simulink library "lib_controller"  (R2015a)
settings: Solver=ode45  StartTime=0.0  StopTime=10.0  RelTol=1e-3
values from neighbouring files (symbols this model uses):
  CG_0 = [0,0,0.02]'    [SetupComplete.m]
  g = 9.81    [SetupComplete.m]
  h_M = 0.064    [SetupComplete.m]
  I_BAC_0 = [ Ix,0,Ixz;0,Iy,0;Ixz,0,Iz]    [SetupComplete.m]
  l = 0.3450    (= 0.345)    [NDI_components.m]    (also in SetupComplete.m; robust_controller.m)
  m = 3.51    [SetupComplete.m]
  m_0 = 2.61    [SetupComplete.m]
  m_M = 0.300    (= 0.3)    [SetupComplete.m]
  T_sim = 0.01    [Run3Copter.m]
undefined symbols (not defined in the file or in its folder): Theta_1_roll_last, Theta_2_roll_last, Theta_3_roll_last, V_long_lastA_w_z, V_long_lastAoA, V_roll_last, V_yaw_last, W_long_lastA_w_z, W_long_lastAoA, W_roll_last, W_yaw_last
libraries: simulink x65, Adaptive_FaultTolerantControl x8, lib_controller x5, qcatlib x4, dspinverses x4, aerolibtransform2 x3, aerolib6dofsys x1
(part 10 of 10)

== matlab function lib_controller/Controller/NDI+CA Controller/9DOF ANN+NDI+CA Controller - No massic update/F(X) 9DOF_UVWPQR ==
  data: fx output size=[6,1]; prev_input input size=[9,1]; gforce_body input size=[3,1]; omega_body input size=[3,1]; v_body input size=[3,1]
function fx = fx(prev_input, gforce_body, omega_body, v_body)
    % Calculates f_hat(x). The expression is calculated in NDI_components
    % x_dot = f(x) + g(x,u)
    %   g(x,u) ~= g(x,u0) + jac(g(x,u), u)(u0) * (u - u0)
    %   g(x,u) ~= h(x,u0) + jac(g(x,u), u)(u0) * u
    % x_dot = f_hat(x) + jac(g(x,u), u) * u
    %   f_hat(x) = f(x) + g(x,u0) - jac(g(x,u), u)(u0) *  u0
    %   g_hat(x) = jac(g(x,u), u)(u0)
    % x_dot = f_hat(x) + g_hat(x) * u
    tau1_0 = prev_input(1);
    eta1_0 = prev_input(2);
    gamma1_0 = prev_input(3);
    tau2_0 = prev_input(4);
    eta2_0 = prev_input(5);
    gamma2_0 = prev_input(6);
    tau3_0 = prev_input(7);
    eta3_0 = prev_input(8);
    gamma3_0 = prev_input(9);
    Gx =  gforce_body(1);
    Gy =  gforce_body(2);
    Gz =  gforce_body(3);
    U = v_body(1);
    V = v_body(2);
    W = v_body(3);
    P = omega_body(1);
    Q = omega_body(2);
    R = omega_body(3);

    % This matrix was precomputed in NDI_components.m
    % TODO Precompute sines and cosines to improve performance. Some
    % repeated terms can also be precomputed
    
 fx = [...
 5.88e-5*P^2 + 0.00285*P*R - 5.88e-5*R^2 + 1.0*V*R + 0.285*Gx - 1.0*Q*W + 4.27*gamma1_0*tau1_0*cos(gamma1_0) + 5.14e-4*gamma2_0*tau2_0*cos(gamma2_0) + 5.14e-4*gamma3_0*tau3_0*cos(gamma3_0) - 5.14e-4*eta1_0*tau1_0*cos(eta1_0)*cos(gamma1_0) + 4.27*eta2_0*tau2_0*cos(eta2_0)*cos(gamma2_0) + 4.27*eta3_0*tau3_0*cos(eta3_0)*cos(gamma3_0) + 0.038*eta1_0*tau1_0*cos(gamma1_0)*sin(eta1_0) - 0.019*eta2_0*tau2_0*cos(gamma2_0)*sin(eta2_0) - 0.019*eta3_0*tau3_0*cos(gamma3_0)*sin(eta3_0) + 0.038*gamma1_0*tau1_0*cos(eta1_0)*sin(gamma1_0) - 0.019*gamma2_0*tau2_0*cos(eta2_0)*sin(gamma2_0) - 0.019*gamma3_0*tau3_0*cos(eta3_0)*sin(gamma3_0) + 5.14e-4*gamma1_0*tau1_0*sin(eta1_0)*sin(gamma1_0) - 4.27*gamma2_0*tau2_0*sin(eta2_0)*sin(gamma2_0) - 4.27*gamma3_0*tau3_0*sin(eta3_0)*sin(gamma3_0);
        0.285*Gy + 6.54e-5*P*Q + 0.00281*Q*R + 1.0*P*W - 1.0*R*U - 6.56e-4*gamma1_0*tau1_0*cos(gamma1_0) - 4.27*gamma2_0*tau2_0*cos(gamma2_0) - 4.27*gamma3_0*tau3_0*cos(gamma3_0) - 4.27*eta1_0*tau1_0*cos(eta1_0)*cos(gamma1_0) - 3.21e-4*eta2_0*tau2_0*cos(eta2_0)*cos(gamma2_0) + 0.00163*eta3_0*tau3_0*cos(eta3_0)*cos(gamma3_0) - 1.53e-5*eta1_0*tau1_0*cos(gamma1_0)*sin(eta1_0) + 0.042*eta2_0*tau2_0*cos(gamma2_0)*sin(eta2_0) - 0.042*eta3_0*tau3_0*cos(gamma3_0)*sin(eta3_0) - 1.53e-5*gamma1_0*tau1_0*cos(eta1_0)*sin(gamma1_0) + 0.042*gamma2_0*tau2_0*cos(eta2_0)*sin(gamma2_0) - 0.042*gamma3_0*tau3_0*cos(eta3_0)*sin(gamma3_0) + 4.27*gamma1_0*tau1_0*sin(eta1_0)*sin(gamma1_0) + 3.21e-4*gamma2_0*tau2_0*sin(eta2_0)*sin(gamma2_0) - 0.00163*gamma3_0*tau3_0*sin(eta3_0)*sin(gamma3_0);
                                                                                                                                                                                                                                                                                                                                                                                                                                                - 0.0015*P^2 - 1.0*V*P - 0.0015*Q^2 + 1.0*U*Q + 0.285*Gz - 4.27*eta1_0*tau1_0*cos(gamma1_0)*sin(eta1_0) - 4.27*eta2_0*tau2_0*cos(gamma2_0)*sin(eta2_0) - 4.27*eta3_0*tau3_0*cos(gamma3_0)*sin(eta3_0) - 4.27*gamma1_0*tau1_0*cos(eta1_0)*sin(gamma1_0) - 4.27*gamma2_0*tau2_0*cos(eta2_0)*sin(gamma2_0) - 4.27*gamma3_0*tau3_0*cos(eta3_0)*sin(gamma3_0);
                                                        0.437*gamma1_0*tau1_0*cos(gamma1_0) - 0.876*Q*R - 0.0436*P*Q - 0.235*gamma2_0*tau2_0*cos(gamma2_0) - 0.235*gamma3_0*tau3_0*cos(gamma3_0) + 0.893*eta1_0*tau1_0*cos(eta1_0)*cos(gamma1_0) + 0.214*eta2_0*tau2_0*cos(eta2_0)*cos(gamma2_0) - 1.09*eta3_0*tau3_0*cos(eta3_0)*cos(gamma3_0) + 0.0102*eta1_0*tau1_0*cos(gamma1_0)*sin(eta1_0) - 28.0*eta2_0*tau2_0*cos(gamma2_0)*sin(eta2_0) + 28.0*eta3_0*tau3_0*cos(gamma3_0)*sin(eta3_0) + 0.0102*gamma1_0*tau1_0*cos(eta1_0)*sin(gamma1_0) - 28.0*gamma2_0*tau2_0*cos(eta2_0)*sin(gamma2_0) + 28.0*gamma3_0*tau3_0*cos(eta3_0)*sin(gamma3_0) - 0.893*gamma1_0*tau1_0*sin(eta1_0)*sin(gamma1_0) - 0.214*gamma2_0*tau2_0*sin(eta2_0)*sin(gamma2_0) + 1.09*gamma3_0*tau3_0*sin(eta3_0)*sin(gamma3_0);
                                                  0.0392*P^2 + 0.901*P*R - 0.0392*R^2 + 0.11*gamma1_0*tau1_0*cos(gamma1_0) + 0.343*gamma2_0*tau2_0*cos(gamma2_0) + 0.343*gamma3_0*tau3_0*cos(gamma3_0) - 0.343*eta1_0*tau1_0*cos(eta1_0)*cos(gamma1_0) + 0.11*eta2_0*tau2_0*cos(eta2_0)*cos(gamma2_0) + 0.11*eta3_0*tau3_0*cos(eta3_0)*cos(gamma3_0) + 25.3*eta1_0*tau1_0*cos(gamma1_0)*sin(eta1_0) - 12.7*eta2_0*tau2_0*cos(gamma2_0)*sin(eta2_0) - 12.7*eta3_0*tau3_0*cos(gamma3_0)*sin(eta3_0) + 25.3*gamma1_0*tau1_0*cos(eta1_0)*sin(gamma1_0) - 12.7*gamma2_0*tau2_0*cos(eta2_0)*sin(gamma2_0) - 12.7*gamma3_0*tau3_0*cos(eta3_0)*sin(gamma3_0) + 0.343*gamma1_0*tau1_0*sin(eta1_0)*sin(gamma1_0) - 0.11*gamma2_0*tau2_0*sin(eta2_0)*sin(gamma2_0) - 0.11*gamma3_0*tau3_0*sin(eta3_0)*sin(gamma3_0);
                                                           0.0436*Q*R - 0.127*P*Q - 0.0102*gamma1_0*tau1_0*cos(gamma1_0) + 7.53*gamma2_0*tau2_0*cos(gamma2_0) + 7.53*gamma3_0*tau3_0*cos(gamma3_0) - 15.1*eta1_0*tau1_0*cos(eta1_0)*cos(gamma1_0) - 13.0*eta2_0*tau2_0*cos(eta2_0)*cos(gamma2_0) + 13.0*eta3_0*tau3_0*cos(eta3_0)*cos(gamma3_0) - 0.204*eta1_0*tau1_0*cos(gamma1_0)*sin(eta1_0) + 0.855*eta2_0*tau2_0*cos(gamma2_0)*sin(eta2_0) - 0.448*eta3_0*tau3_0*cos(gamma3_0)*sin(eta3_0) - 0.204*gamma1_0*tau1_0*cos(eta1_0)*sin(gamma1_0) + 0.855*gamma2_0*tau2_0*cos(eta2_0)*sin(gamma2_0) - 0.448*gamma3_0*tau3_0*cos(eta3_0)*sin(gamma3_0) + 15.1*gamma1_0*tau1_0*sin(eta1_0)*sin(gamma1_0) + 13.0*gamma2_0*tau2_0*sin(eta2_0)*sin(gamma2_0) - 13.0*gamma3_0*tau3_0*sin(eta3_0)*sin(gamma3_0)];

== matlab function lib_controller/Controller/NDI+CA Controller/9DOF ANN+NDI+CA Controller - No massic update/G(X) 9DOF_UVWPQR ==
  data: gx output size=[6,9]; prev_input input size=[9,1]
function gx = gx(prev_input)
    % Calculates f_hat(x). The expression is calculated in NDI_components
    % x_dot = f(x) + g(x,u)
    %   g(x,u) ~= g(x,u0) + jac(g(x,u), u)(u0) * (u - u0)
    %   g(x,u) ~= h(x,u0) + jac(g(x,u), u)(u0) * u
    % x_dot = f_hat(x) + jac(g(x,u), u) * u
    %   f_hat(x) = f(x) + g(x,u0) - jac(g(x,u), u)(u0) *  u0
    %   g_hat(x) = jac(g(x,u), u)(u0)
    % x_dot = f_hat(x) + g_hat(x) * u
    tau1_0 = prev_input(1);
    eta1_0 = prev_input(2);
    gamma1_0 = prev_input(3);
    tau2_0 = prev_input(4);
    eta2_0 = prev_input(5);
    gamma2_0 = prev_input(6);
    tau3_0 = prev_input(7);
    eta3_0 = prev_input(8);
    gamma3_0 = prev_input(9);
    
    % This matrix was precomputed in NDI_components.m
    % TODO Precompute sines and cosines to improve performance. Some
    % repeated terms can also be precomputed
    gx = [...
   5.14e-4*cos(gamma1_0)*sin(eta1_0) - 4.27*sin(gamma1_0) + 0.038*cos(eta1_0)*cos(gamma1_0),  5.14e-4*tau1_0*cos(eta1_0)*cos(gamma1_0) - 0.038*tau1_0*cos(gamma1_0)*sin(eta1_0), - 4.27*tau1_0*cos(gamma1_0) - 0.038*tau1_0*cos(eta1_0)*sin(gamma1_0) - 5.14e-4*tau1_0*sin(eta1_0)*sin(gamma1_0), - 5.14e-4*sin(gamma2_0) - 4.27*cos(gamma2_0)*sin(eta2_0) - 0.019*cos(eta2_0)*cos(gamma2_0),    0.019*tau2_0*cos(gamma2_0)*sin(eta2_0) - 4.27*tau2_0*cos(eta2_0)*cos(gamma2_0), 0.019*tau2_0*cos(eta2_0)*sin(gamma2_0) - 5.14e-4*tau2_0*cos(gamma2_0) + 4.27*tau2_0*sin(eta2_0)*sin(gamma2_0), - 5.14e-4*sin(gamma3_0) - 4.27*cos(gamma3_0)*sin(eta3_0) - 0.019*cos(eta3_0)*cos(gamma3_0),    0.019*tau3_0*cos(gamma3_0)*sin(eta3_0) - 4.27*tau3_0*cos(eta3_0)*cos(gamma3_0), 0.019*tau3_0*cos(eta3_0)*sin(gamma3_0) - 5.14e-4*tau3_0*cos(gamma3_0) + 4.27*tau3_0*sin(eta3_0)*sin(gamma3_0);
 6.56e-4*sin(gamma1_0) + 4.27*cos(gamma1_0)*sin(eta1_0) - 1.53e-5*cos(eta1_0)*cos(gamma1_0),   4.27*tau1_0*cos(eta1_0)*cos(gamma1_0) + 1.53e-5*tau1_0*cos(gamma1_0)*sin(eta1_0), 6.56e-4*tau1_0*cos(gamma1_0) + 1.53e-5*tau1_0*cos(eta1_0)*sin(gamma1_0) - 4.27*tau1_0*sin(eta1_0)*sin(gamma1_0),   4.27*sin(gamma2_0) + 3.21e-4*cos(gamma2_0)*sin(eta2_0) + 0.042*cos(eta2_0)*cos(gamma2_0), 3.21e-4*tau2_0*cos(eta2_0)*cos(gamma2_0) - 0.042*tau2_0*cos(gamma2_0)*sin(eta2_0), 4.27*tau2_0*cos(gamma2_0) - 0.042*tau2_0*cos(eta2_0)*sin(gamma2_0) - 3.21e-4*tau2_0*sin(eta2_0)*sin(gamma2_0),   4.27*sin(gamma3_0) - 0.00163*cos(gamma3_0)*sin(eta3_0) - 0.042*cos(eta3_0)*cos(gamma3_0), 0.042*tau3_0*cos(gamma3_0)*sin(eta3_0) - 0.00163*tau3_0*cos(eta3_0)*cos(gamma3_0), 4.27*tau3_0*cos(gamma3_0) + 0.042*tau3_0*cos(eta3_0)*sin(gamma3_0) + 0.00163*tau3_0*sin(eta3_0)*sin(gamma3_0);
                                                            -4.27*cos(eta1_0)*cos(gamma1_0),                                              4.27*tau1_0*cos(gamma1_0)*sin(eta1_0),                                                                           4.27*tau1_0*cos(eta1_0)*sin(gamma1_0),                                                            -4.27*cos(eta2_0)*cos(gamma2_0),                                             4.27*tau2_0*cos(gamma2_0)*sin(eta2_0),                                                                         4.27*tau2_0*cos(eta2_0)*sin(gamma2_0),                                                            -4.27*cos(eta3_0)*cos(gamma3_0),                                             4.27*tau3_0*cos(gamma3_0)*sin(eta3_0),                                                                         4.27*tau3_0*cos(eta3_0)*sin(gamma3_0);
   0.0102*cos(eta1_0)*cos(gamma1_0) - 0.893*cos(gamma1_0)*sin(eta1_0) - 0.437*sin(gamma1_0), - 0.893*tau1_0*cos(eta1_0)*cos(gamma1_0) - 0.0102*tau1_0*cos(gamma1_0)*sin(eta1_0),   0.893*tau1_0*sin(eta1_0)*sin(gamma1_0) - 0.0102*tau1_0*cos(eta1_0)*sin(gamma1_0) - 0.437*tau1_0*cos(gamma1_0),     0.235*sin(gamma2_0) - 0.214*cos(gamma2_0)*sin(eta2_0) - 28.0*cos(eta2_0)*cos(gamma2_0),    28.0*tau2_0*cos(gamma2_0)*sin(eta2_0) - 0.214*tau2_0*cos(eta2_0)*cos(gamma2_0),   0.235*tau2_0*cos(gamma2_0) + 28.0*tau2_0*cos(eta2_0)*sin(gamma2_0) + 0.214*tau2_0*sin(eta2_0)*sin(gamma2_0),      0.235*sin(gamma3_0) + 1.09*cos(gamma3_0)*sin(eta3_0) + 28.0*cos(eta3_0)*cos(gamma3_0),     1.09*tau3_0*cos(eta3_0)*cos(gamma3_0) - 28.0*tau3_0*cos(gamma3_0)*sin(eta3_0),    0.235*tau3_0*cos(gamma3_0) - 28.0*tau3_0*cos(eta3_0)*sin(gamma3_0) - 1.09*tau3_0*sin(eta3_0)*sin(gamma3_0);
      0.343*cos(gamma1_0)*sin(eta1_0) - 0.11*sin(gamma1_0) + 25.3*cos(eta1_0)*cos(gamma1_0),     0.343*tau1_0*cos(eta1_0)*cos(gamma1_0) - 25.3*tau1_0*cos(gamma1_0)*sin(eta1_0),    - 0.11*tau1_0*cos(gamma1_0) - 25.3*tau1_0*cos(eta1_0)*sin(gamma1_0) - 0.343*tau1_0*sin(eta1_0)*sin(gamma1_0),    - 0.343*sin(gamma2_0) - 0.11*cos(gamma2_0)*sin(eta2_0) - 12.7*cos(eta2_0)*cos(gamma2_0),     12.7*tau2_0*cos(gamma2_0)*sin(eta2_0) - 0.11*tau2_0*cos(eta2_0)*cos(gamma2_0),    12.7*tau2_0*cos(eta2_0)*sin(gamma2_0) - 0.343*tau2_0*cos(gamma2_0) + 0.11*tau2_0*sin(eta2_0)*sin(gamma2_0),    - 0.343*sin(gamma3_0) - 0.11*cos(gamma3_0)*sin(eta3_0) - 12.7*cos(eta3_0)*cos(gamma3_0),     12.7*tau3_0*cos(gamma3_0)*sin(eta3_0) - 0.11*tau3_0*cos(eta3_0)*cos(gamma3_0),    12.7*tau3_0*cos(eta3_0)*sin(gamma3_0) - 0.343*tau3_0*cos(gamma3_0) + 0.11*tau3_0*sin(eta3_0)*sin(gamma3_0);
    0.0102*sin(gamma1_0) + 15.1*cos(gamma1_0)*sin(eta1_0) - 0.204*cos(eta1_0)*cos(gamma1_0),     15.1*tau1_0*cos(eta1_0)*cos(gamma1_0) + 0.204*tau1_0*cos(gamma1_0)*sin(eta1_0),    0.0102*tau1_0*cos(gamma1_0) + 0.204*tau1_0*cos(eta1_0)*sin(gamma1_0) - 15.1*tau1_0*sin(eta1_0)*sin(gamma1_0),      13.0*cos(gamma2_0)*sin(eta2_0) - 7.53*sin(gamma2_0) + 0.855*cos(eta2_0)*cos(gamma2_0),    13.0*tau2_0*cos(eta2_0)*cos(gamma2_0) - 0.855*tau2_0*cos(gamma2_0)*sin(eta2_0),  - 7.53*tau2_0*cos(gamma2_0) - 0.855*tau2_0*cos(eta2_0)*sin(gamma2_0) - 13.0*tau2_0*sin(eta2_0)*sin(gamma2_0),    - 7.53*sin(gamma3_0) - 13.0*cos(gamma3_0)*sin(eta3_0) - 0.448*cos(eta3_0)*cos(gamma3_0),    0.448*tau3_0*cos(gamma3_0)*sin(eta3_0) - 13.0*tau3_0*cos(eta3_0)*cos(gamma3_0),    0.448*tau3_0*cos(eta3_0)*sin(gamma3_0) - 7.53*tau3_0*cos(gamma3_0) + 13.0*tau3_0*sin(eta3_0)*sin(gamma3_0)];
 
    
    
    
    
%  0.038016*cos(eta1_0) + 0.00051422*sin(eta1_0), 0.00051422*tau1_0*cos(eta1_0) - 0.038016*tau1_0*sin(eta1_0),    -4.2737*tau1_0, -0.019008,    -4.2737*tau2_0, -0.00051422*tau2_0, -0.019008,   -4.2737*tau3_0, -0.00051422*tau3_0;
%   4.2748*sin(eta1_0) - 0.000015257*cos(eta1_0),  4.2748*tau1_0*cos(eta1_0) + 0.000015257*tau1_0*sin(eta1_0), 0.00065622*tau1_0,  0.042029, 0.00032056*tau2_0,      4.2732*tau2_0, -0.041999, -0.001633*tau3_0,      4.2732*tau3_0;
%                            -4.2735*cos(eta1_0),                                   4.2735*tau1_0*sin(eta1_0),                 0,   -4.2735,                 0,                  0,   -4.2735,                0,                  0;
%     0.010171*cos(eta1_0) - 0.89255*sin(eta1_0),  - 0.89255*tau1_0*cos(eta1_0) - 0.010171*tau1_0*sin(eta1_0),   -0.43748*tau1_0,    -28.02,   -0.21371*tau2_0,     0.23535*tau2_0,    27.999,    1.0887*tau3_0,     0.23535*tau3_0;
%       25.344*cos(eta1_0) + 0.34281*sin(eta1_0),      0.34281*tau1_0*cos(eta1_0) - 25.344*tau1_0*sin(eta1_0),   -0.11019*tau1_0,   -12.672,   -0.11019*tau2_0,    -0.34281*tau2_0,   -12.672,  -0.11019*tau3_0,    -0.34281*tau3_0;
%        15.06*sin(eta1_0) - 0.20367*cos(eta1_0),       15.06*tau1_0*cos(eta1_0) + 0.20367*tau1_0*sin(eta1_0),   0.010171*tau1_0,   0.85486,     13.029*tau2_0,     -7.5251*tau2_0,  -0.44753,    -13.05*tau3_0,     -7.5251*tau3_0];

== matlab function lib_controller/Controller/NDI+CA Controller/9DOF ANN+NDI+CA Controller - No massic update/Rotational Kinematics ==
  data: PQR output size=3; Eulerdot input size=3; Euler input size=3
function PQR = rot_kin(Eulerdot,Euler)
%solves rotational kinematic equations
Phi = Euler(1);
Theta = Euler(2);
Psi = Euler(3);
A = [1 sin(Phi)*tan(Theta) cos(Phi)*tan(Theta);
     0 cos(Phi) -sin(Phi);
     0 sin(Phi)*sec(Theta) cos(Phi)*sec(Theta)];
PQR = A'*Eulerdot;
end

== matlab function lib_controller/Controller/NDI+CA Controller/9DOF ANN+NDI+CA Controller - No massic update/Rotational Kinematics1 ==
  data: PQR input size=3; Eulerdot output size=3; Euler input size=3
function Eulerdot = rot_kin(PQR,Euler)
%solves rotational kinematic equations
Phi = Euler(1);
Theta = Euler(2);
Psi = Euler(3);
A = [1 sin(Phi)*tan(Theta) cos(Phi)*tan(Theta);
     0 cos(Phi) -sin(Phi);
     0 sin(Phi)*sec(Theta) cos(Phi)*sec(Theta)];
Eulerdot = A*PQR;
end

== matlab function lib_controller/Controller/NDI+CA Controller/9DOF ANN+NDI+CA Controller - No massic update/Rotational Kinematics2 ==
  data: PQR output size=3; Eulerdot input size=3; Euler input size=3
function PQR = rot_kin(Eulerdot,Euler)
%solves rotational kinematic equations
Phi = Euler(1);
Theta = Euler(2);
Psi = Euler(3);
A = [1 sin(Phi)*tan(Theta) cos(Phi)*tan(Theta);
     0 cos(Phi) -sin(Phi);
     0 sin(Phi)*sec(Theta) cos(Phi)*sec(Theta)];
PQR = A'*Eulerdot;
end

== matlab function lib_controller/Controller/NDI+CA Controller/9DOF ANN+NDI+CA Controller - No massic update/Sigmoid /MATLAB Function ==
  data: u input; y output; a input
function y = sigmoid_a(u,a)

y = 2.0 ./ (1.0 + exp(-a*u(:)))-1;
